simulink model "DAL_Sat_SW"  (R2021b)
settings: Solver=FixedStepAuto  StartTime=0.0  StopTime=Inf  RelTol=1e-3  EnableMultiTasking=on
undefined symbols (not defined in the file): Beam_Mod, magnitude, N_B
settings Model: ExtModeTrigDuration=2  Creator=diego  LastModifiedBy=diego
settings OptimizationCC: EnhancedBackFolding=on  PassReuseOutputArgsAs=Individual arguments  ZeroExternalMemoryAtStartup=off  ZeroInternalMemoryAtStartup=off  MaxStackSize=64  OptimizeBlockOrder=speed  DifferentSizesBufferReuse=on  EfficientTunableParamExpr=on
settings DebuggingCC: ParameterTunabilityLossMsg=error
settings HardwareCC: ProdBitPerInt=16  ProdBitPerPointer=16  ProdBitPerSizeT=16  ProdBitPerPtrDiffT=16  ProdLargestAtomicFloat=None  ProdWordSize=8  ProdHWDeviceType=Atmel->AVR
settings SFSimCC: MATLABDynamicMemAlloc=off
settings RTWCC: Description=Embedded Coder  SystemTargetFile=ert.tlc  HardwareBoard=Arduino Uno  TemplateMakefile=ert_default_tmf  Toolchain=Arduino AVR  BuildConfiguration=Faster Runs
settings CodeAppCC: ForceParamTrailComments=on  IgnoreCustomStorageClasses=off  OperatorAnnotations=on  SimulinkDataObjDesc=on  SFDataObjDesc=on  InsertBlockDesc=on
settings ERTTargetCC: SupportContinuousTime=on  SupportVariableSizeSignals=on  ExtModeTransport=3  ExtModeStaticAlloc=on  ExtModeStaticAllocSize=250  ExtModeMexFile=ext_xcp  ExtModeIntrfLevel=Level2 - Open

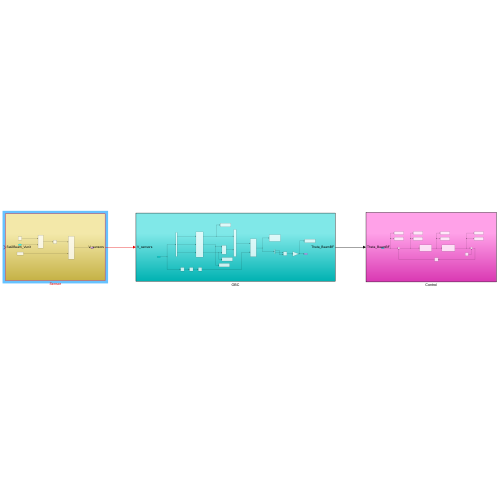
[thumbnail: Simulink's stored preview of the top-level diagram]
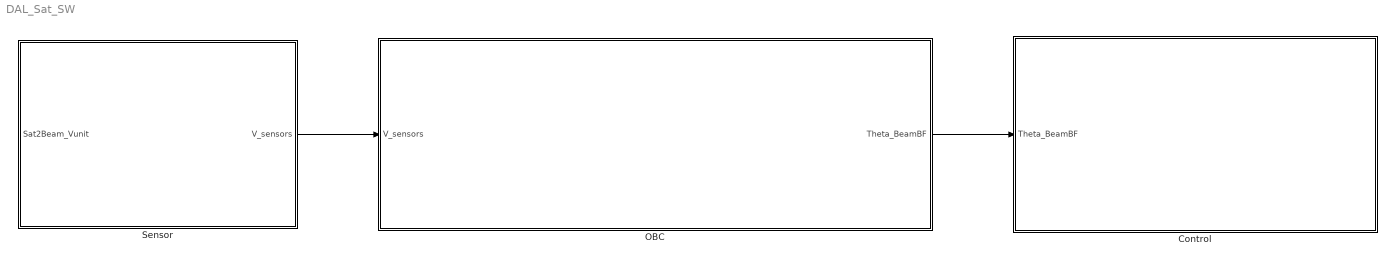
== system DAL_Sat_SW ==
  Control : Subsystem
  OBC : Subsystem
  Sensor : Subsystem
  wires:
  OBC/1(Theta_BeamBF) -> Control/1(Theta_BeamBF)
  Sensor/1(V_sensors) -> OBC/1(V_sensors)

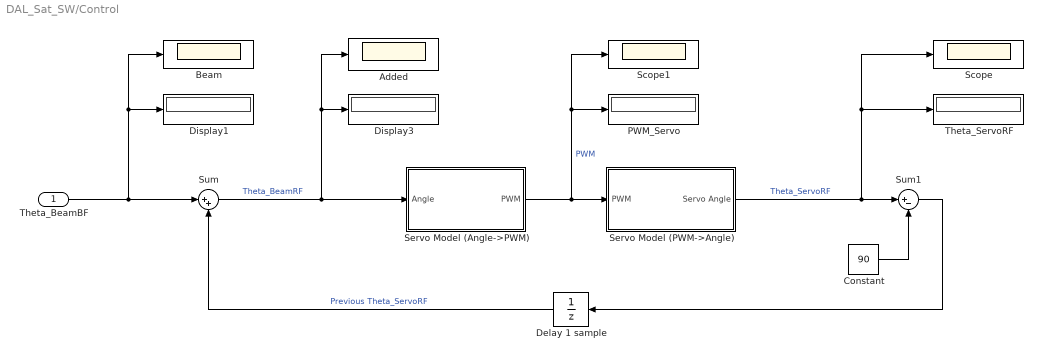
== system DAL_Sat_SW/Control ==
  Theta_BeamBF : Inport
  Added : Scope
  Beam : Scope
  Constant : Constant  Value=90
  Delay 1 sample : UnitDelay  SampleTime=-1  HasFrameUpgradeWarning=on
  Display1 : Display
  Display3 : Display
  PWM_Servo : Display
  Scope : Scope
  Scope1 : Scope
  Servo Model (Angle->PWM) : Subsystem
  Servo Model (PWM->Angle) : Subsystem
  Sum : Sum  Inputs=|++
  Sum1 : Sum  Inputs=|+-
  Theta_ServoRF : Display
  wires:
  Servo Model (PWM->Angle)/1(Servo Angle) -> Theta_ServoRF/1, Scope/1, Sum1/1  "Theta_ServoRF"
  Delay 1 sample/1 -> Sum/2  "Previous Theta_ServoRF"
  Theta_BeamBF/1 -> Sum/1, Beam/1, Display1/1
  Sum1/1 -> Delay 1 sample/1
  Constant/1 -> Sum1/2
  Sum/1 -> Servo Model (Angle->PWM)/1(Angle), Added/1, Display3/1  "Theta_BeamRF"
  Servo Model (Angle->PWM)/1(PWM) -> Scope1/1, PWM_Servo/1, Servo Model (PWM->Angle)/1(PWM)  "PWM"

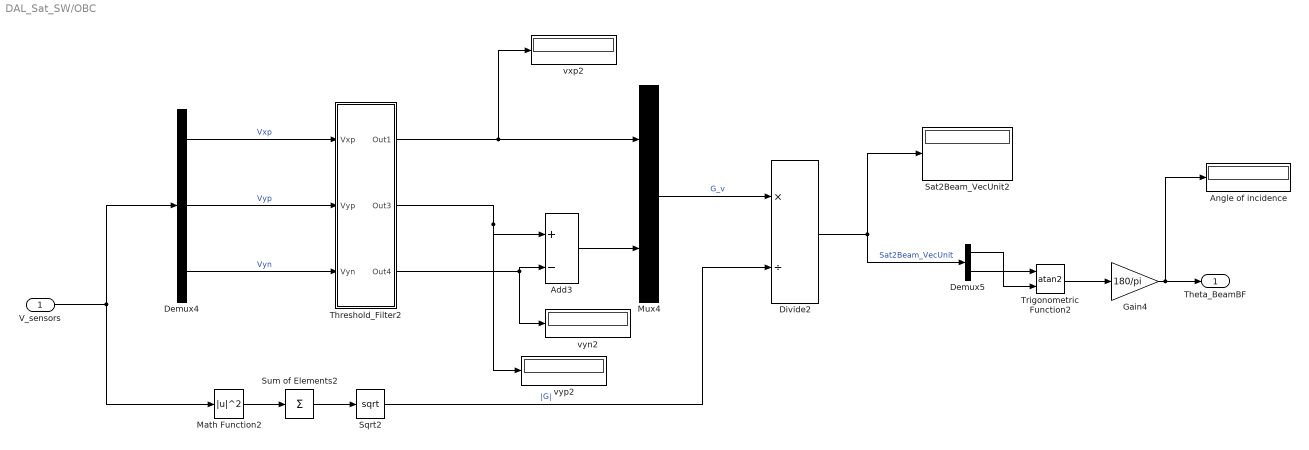
== system DAL_Sat_SW/OBC ==
  V_sensors : Inport
  Add3 : Sum  Inputs=+|-
  Angle of incidence : Display
  Demux4 : Demux  Outputs=3
  Demux5 : Demux  Outputs=2
  Divide2 : Product  Inputs=*/
  Gain4 : Gain  Gain=180/pi
  Math Function2 : Math  Operator=magnitude^2  OutputSignalType=real  SaturateOnIntegerOverflow=on
  Mux4 : Mux  Inputs=2
  Sat2Beam_VecUnit2 : Display
  Sqrt2 : Sqrt  SaturateOnIntegerOverflow=on
  Sum of Elements2 : Sum  Inputs=+
  Threshold_Filter2 : Subsystem
  Trigonometric Function2 : Trigonometry  Operator=atan2
  vxp2 : Display
  vyn2 : Display
  vyp2 : Display
  Theta_BeamBF : Outport
  wires:
  V_sensors/1 -> Demux4/1, Math Function2/1
  Demux4/2 -> Threshold_Filter2/2(Vyp)  "Vyp"
  Trigonometric Function2/1 -> Gain4/1
  Threshold_Filter2/1(Out1) -> vxp2/1, Mux4/1
  Divide2/1 -> Demux5/1, Sat2Beam_VecUnit2/1  "Sat2Beam_VecUnit"
  Demux4/3 -> Threshold_Filter2/3(Vyn)  "Vyn"
  Sqrt2/1 -> Divide2/2  "|G|"
  Demux5/1 -> Trigonometric Function2/2
  Demux4/1 -> Threshold_Filter2/1(Vxp)  "Vxp"
  Threshold_Filter2/3(Out4) -> vyn2/1, Add3/2
  Add3/1 -> Mux4/2
  Threshold_Filter2/2(Out3) -> vyp2/1, Add3/1
  Mux4/1 -> Divide2/1  "G_v"
  Demux5/2 -> Trigonometric Function2/1
  Sum of Elements2/1 -> Sqrt2/1
  Math Function2/1 -> Sum of Elements2/1
  Gain4/1 -> Angle of incidence/1, Theta_BeamBF/1

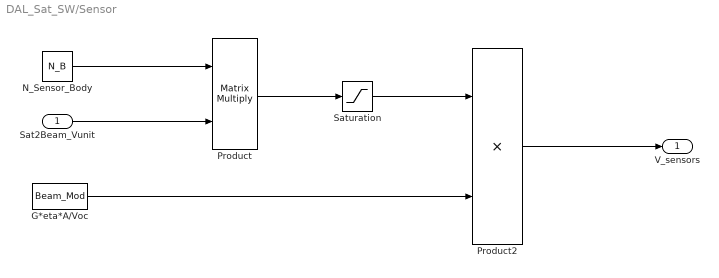
== system DAL_Sat_SW/Sensor ==
  Sat2Beam_Vunit : Inport
  G*eta*A/Voc : Constant  Value=Beam_Mod
  N_Sensor_Body : Constant  Value=N_B
  Product : Product  Multiplication=Matrix(*)
  Product2 : Product
  Saturation : Saturate  UpperLimit=1  LowerLimit=0
  V_sensors : Outport
  wires:
  Product/1 -> Saturation/1
  N_Sensor_Body/1 -> Product/1
  Saturation/1 -> Product2/1
  Product2/1 -> V_sensors/1
  Sat2Beam_Vunit/1 -> Product/2
  G*eta*A/Voc/1 -> Product2/2

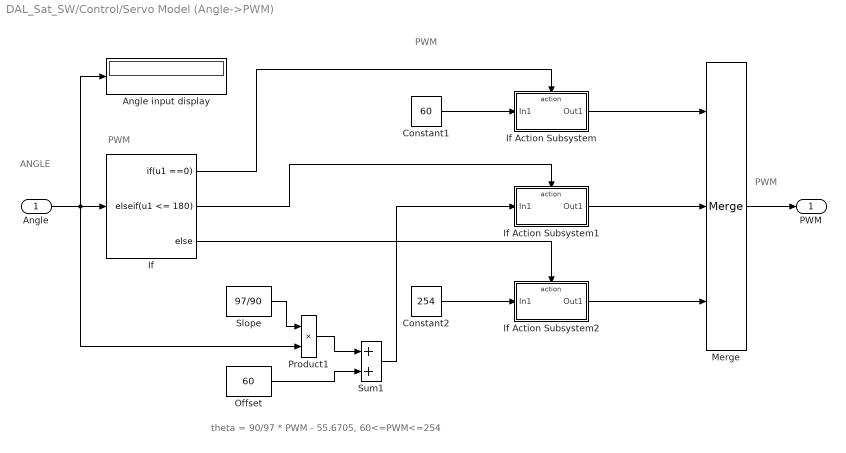
== system DAL_Sat_SW/Control/Servo Model (Angle->PWM) ==
  note: PWM
  note: ANGLE
  note: PWM
  note: PWM
  note: theta = 90/97 * PWM - 55.6705, 60<=PWM<=254
  Angle : Inport
  Angle input display : Display
  Constant1 : Constant  Value=60
  Constant2 : Constant  Value=254
  If : If  IfExpression=u1 ==0  ElseIfExpressions=u1 <= 180
  If Action Subsystem : Subsystem  TreatAsAtomicUnit=on
  If Action Subsystem1 : Subsystem  TreatAsAtomicUnit=on
  If Action Subsystem2 : Subsystem  TreatAsAtomicUnit=on
  Merge : Merge  Inputs=3
  Offset : Constant  Value=60
  Product1 : Product
  Slope : Constant  Value=97/90
  Sum1 : Sum
  PWM : Outport
  wires:
  Merge/1 -> PWM/1
  If/2 -> If Action Subsystem1/Action
  Constant1/1 -> If Action Subsystem/1(In1)
  Constant2/1 -> If Action Subsystem2/1(In1)
  If Action Subsystem1/1(Out1) -> Merge/2
  If Action Subsystem2/1(Out1) -> Merge/3
  Slope/1 -> Product1/1
  Sum1/1 -> If Action Subsystem1/1(In1)
  If/1 -> If Action Subsystem/Action
  Angle/1 -> If/1, Angle input display/1, Product1/2
  Product1/1 -> Sum1/1
  If/3 -> If Action Subsystem2/Action
  Offset/1 -> Sum1/2
  If Action Subsystem/1(Out1) -> Merge/1

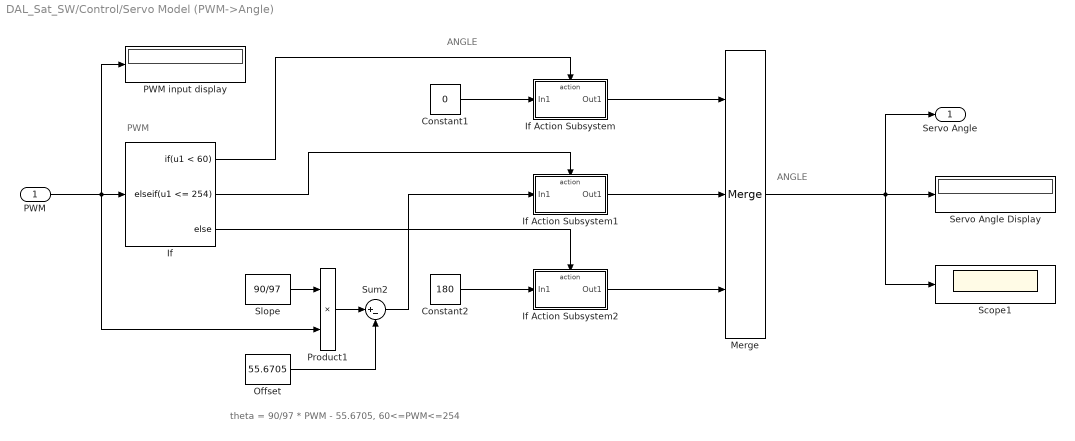
== system DAL_Sat_SW/Control/Servo Model (PWM->Angle) ==
  note: theta = 90/97 * PWM - 55.6705, 60<=PWM<=254
  note: PWM
  note: ANGLE
  note: ANGLE
  PWM : Inport
  Constant1 : Constant  Value=0
  Constant2 : Constant  Value=180
  If : If  IfExpression=u1 < 60  ElseIfExpressions=u1 <= 254
  If Action Subsystem : Subsystem  TreatAsAtomicUnit=on
  If Action Subsystem1 : Subsystem  TreatAsAtomicUnit=on
  If Action Subsystem2 : Subsystem  TreatAsAtomicUnit=on
  Merge : Merge  Inputs=3
  Offset : Constant  Value=55.6705
  PWM input display : Display
  Product1 : Product
  Scope1 : Scope
  Servo Angle Display : Display
  Slope : Constant  Value=90/97
  Sum2 : Sum  Inputs=|+-
  Servo Angle : Outport
  wires:
  Sum2/1 -> If Action Subsystem1/1(In1)
  Slope/1 -> Product1/1
  PWM/1 -> Product1/2, If/1, PWM input display/1
  If/3 -> If Action Subsystem2/Action
  Constant1/1 -> If Action Subsystem/1(In1)
  If Action Subsystem/1(Out1) -> Merge/1
  Merge/1 -> Servo Angle/1, Servo Angle Display/1, Scope1/1
  If Action Subsystem2/1(Out1) -> Merge/3
  Constant2/1 -> If Action Subsystem2/1(In1)
  Product1/1 -> Sum2/1
  If/1 -> If Action Subsystem/Action
  Offset/1 -> Sum2/2
  If Action Subsystem1/1(Out1) -> Merge/2
  If/2 -> If Action Subsystem1/Action

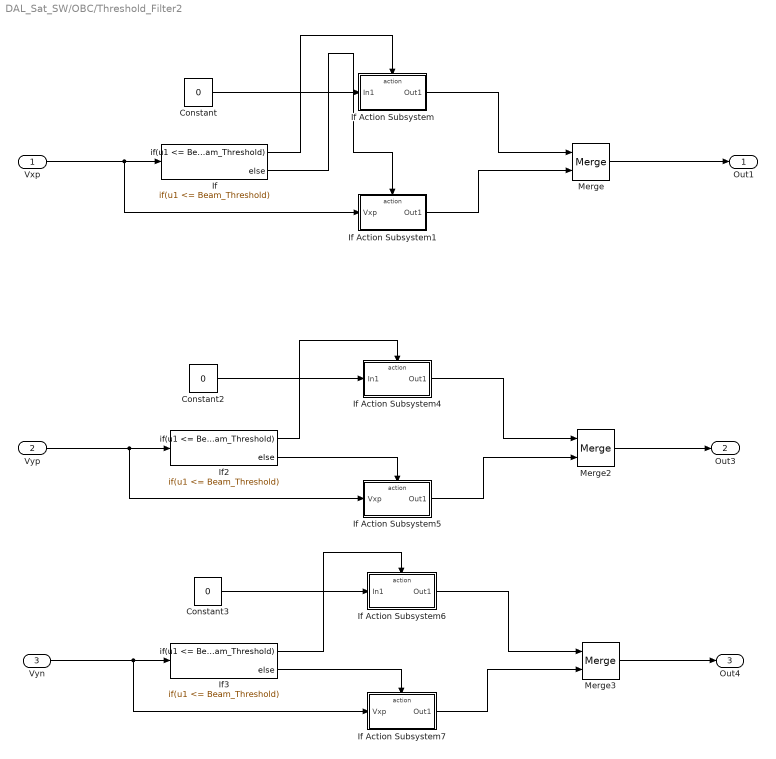
== system DAL_Sat_SW/OBC/Threshold_Filter2 ==
  Vxp : Inport
  Vyp : Inport  Port=2
  Vyn : Inport  Port=3
  Constant : Constant  Value=0
  Constant2 : Constant  Value=0
  Constant3 : Constant  Value=0
  If : If  IfExpression=u1 <= Beam_Threshold
  If Action Subsystem : Subsystem  TreatAsAtomicUnit=on
  If Action Subsystem1 : Subsystem  TreatAsAtomicUnit=on
  If Action Subsystem4 : Subsystem  TreatAsAtomicUnit=on
  If Action Subsystem5 : Subsystem  TreatAsAtomicUnit=on
  If Action Subsystem6 : Subsystem  TreatAsAtomicUnit=on
  If Action Subsystem7 : Subsystem  TreatAsAtomicUnit=on
  If2 : If  IfExpression=u1 <= Beam_Threshold
  If3 : If  IfExpression=u1 <= Beam_Threshold
  Merge : Merge
  Merge2 : Merge
  Merge3 : Merge
  Out1 : Outport
  Out3 : Outport  Port=2
  Out4 : Outport  Port=3
  wires:
  Vxp/1 -> If Action Subsystem1/1(Vxp), If/1
  If/1 -> If Action Subsystem/Action
  If Action Subsystem/1(Out1) -> Merge/1
  If/2 -> If Action Subsystem1/Action
  If Action Subsystem1/1(Out1) -> Merge/2
  Merge/1 -> Out1/1
  Constant/1 -> If Action Subsystem/1(In1)
  Vyp/1 -> If2/1, If Action Subsystem5/1(Vxp)
  If2/2 -> If Action Subsystem5/Action
  If2/1 -> If Action Subsystem4/Action
  If Action Subsystem4/1(Out1) -> Merge2/1
  If Action Subsystem5/1(Out1) -> Merge2/2
  Constant2/1 -> If Action Subsystem4/1(In1)
  Merge2/1 -> Out3/1
  Vyn/1 -> If3/1, If Action Subsystem7/1(Vxp)
  Merge3/1 -> Out4/1
  If Action Subsystem7/1(Out1) -> Merge3/2
  If3/2 -> If Action Subsystem7/Action
  If Action Subsystem6/1(Out1) -> Merge3/1
  Constant3/1 -> If Action Subsystem6/1(In1)
  If3/1 -> If Action Subsystem6/Action

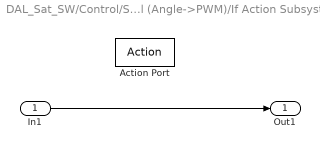
== system DAL_Sat_SW/Control/Servo Model (Angle->PWM)/If Action Subsystem ==
  In1 : Inport
  Action Port : ActionPort
  Out1 : Outport
  wires:
  In1/1 -> Out1/1

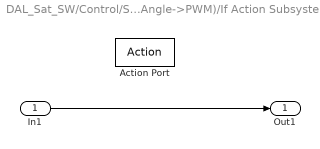
== system DAL_Sat_SW/Control/Servo Model (Angle->PWM)/If Action Subsystem1 ==
  In1 : Inport
  Action Port : ActionPort
  Out1 : Outport
  wires:
  In1/1 -> Out1/1

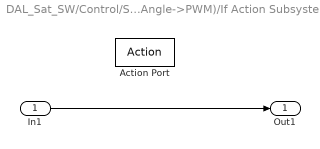
== system DAL_Sat_SW/Control/Servo Model (Angle->PWM)/If Action Subsystem2 ==
  In1 : Inport
  Action Port : ActionPort
  Out1 : Outport
  wires:
  In1/1 -> Out1/1

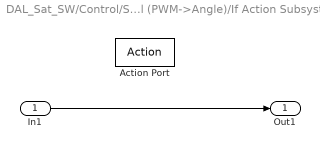
== system DAL_Sat_SW/Control/Servo Model (PWM->Angle)/If Action Subsystem ==
  In1 : Inport
  Action Port : ActionPort  ActionPortLabel=if(u1 < 60)
  Out1 : Outport
  wires:
  In1/1 -> Out1/1

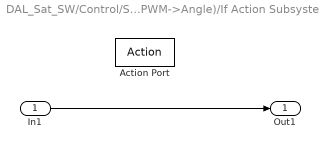
== system DAL_Sat_SW/Control/Servo Model (PWM->Angle)/If Action Subsystem1 ==
  In1 : Inport
  Action Port : ActionPort  ActionPortLabel=elseif(u1 <= 254)
  Out1 : Outport
  wires:
  In1/1 -> Out1/1

== system DAL_Sat_SW/Control/Servo Model (PWM->Angle)/If Action Subsystem2 ==
  In1 : Inport
  Action Port : ActionPort  ActionPortLabel=else
  Out1 : Outport
  wires:
  In1/1 -> Out1/1

== system DAL_Sat_SW/OBC/Threshold_Filter2/If Action Subsystem ==
  In1 : Inport
  Action Port : ActionPort  ActionPortLabel=if(u1 <= Beam_Threshold)
  Out1 : Outport
  wires:
  In1/1 -> Out1/1

== system DAL_Sat_SW/OBC/Threshold_Filter2/If Action Subsystem1 ==
  Vxp : Inport
  Action Port : ActionPort  ActionPortLabel=else
  Out1 : Outport
  wires:
  Vxp/1 -> Out1/1

== system DAL_Sat_SW/OBC/Threshold_Filter2/If Action Subsystem4 ==
  In1 : Inport
  Action Port : ActionPort  ActionPortLabel=if(u1 <= Beam_Threshold)
  Out1 : Outport
  wires:
  In1/1 -> Out1/1

== system DAL_Sat_SW/OBC/Threshold_Filter2/If Action Subsystem5 ==
  Vxp : Inport
  Action Port : ActionPort  ActionPortLabel=else
  Out1 : Outport
  wires:
  Vxp/1 -> Out1/1

== system DAL_Sat_SW/OBC/Threshold_Filter2/If Action Subsystem6 ==
  In1 : Inport
  Action Port : ActionPort  ActionPortLabel=if(u1 <= Beam_Threshold)
  Out1 : Outport
  wires:
  In1/1 -> Out1/1

== system DAL_Sat_SW/OBC/Threshold_Filter2/If Action Subsystem7 ==
  Vxp : Inport
  Action Port : ActionPort  ActionPortLabel=else
  Out1 : Outport
  wires:
  Vxp/1 -> Out1/1
